simulink model "tesys"  (R2021b)
settings: Solver=ode45  StartTime=0  StopTime=inf  FixedStep=1000  RelTol=1e-3  EnableMultiTasking=on
settings Model: PauseTimes=0.0  Creator=ricker  LastModifiedBy=abbas
settings SolverCC: AlgebraicLoopSolver=TrustRegion
settings DataIOCC: LimitDataPoints=on  SaveFormat=Array  SignalLoggingSaveFormat=ModelDataLogs  ReturnWorkspaceOutputs=off  SignalLoggingName=sigsOut
settings OptimizationCC: LifeSpan=inf
settings DebuggingCC: SaveWithParameterizedLinksMsg=none  UnderspecifiedInitializationDetection=Classic  MergeDetectMultiDrivingBlocksExec=none  SignalResolutionControl=TryResolveAllWithWarning  MultiTaskDSMMsg=warning  MultiTaskCondExecSysMsg=none  SFUnexpectedBacktrackingDiag=warning  SFNoUnconditionalDefaultTransitionDiag=warning  SFExecutionAtInitializationDiag=none  SFMachineParentedDataDiag=warning  ArithmeticOperatorsInVariantConditions=warning
settings HardwareCC: ProdBitPerPointer=32  ProdBitPerSizeT=32  ProdBitPerPtrDiffT=32  ProdLargestAtomicFloat=None  ProdIntDivRoundTo=Undefined  ProdEndianess=Unspecified  ProdWordSize=32  ProdHWDeviceType=32-bit Generic  TargetUnknown=on
settings ModelReferenceCC: PropagateSignalLabelsOutOfModel=off
settings SFSimCC: SimUseLocalCustomCode=off  CustomCodeUndefinedFunction=UseInterfaceOnly
settings RTWCC: RTWUseLocalCustomCode=off
settings CodeAppCC: StateflowObjectComments=on
settings GRTTargetCC: TargetLangStandard=C89/C90 (ANSI)  CombineOutputUpdateFcns=off  GRTInterface=on
settings ConfigComp: CovMetricSettings=dw  CovSaveCumulativeToWorkspaceVar=on  CovSaveSingleToWorkspaceVar=on  CovExternalEMLEnable=off  CovSFcnEnable=off

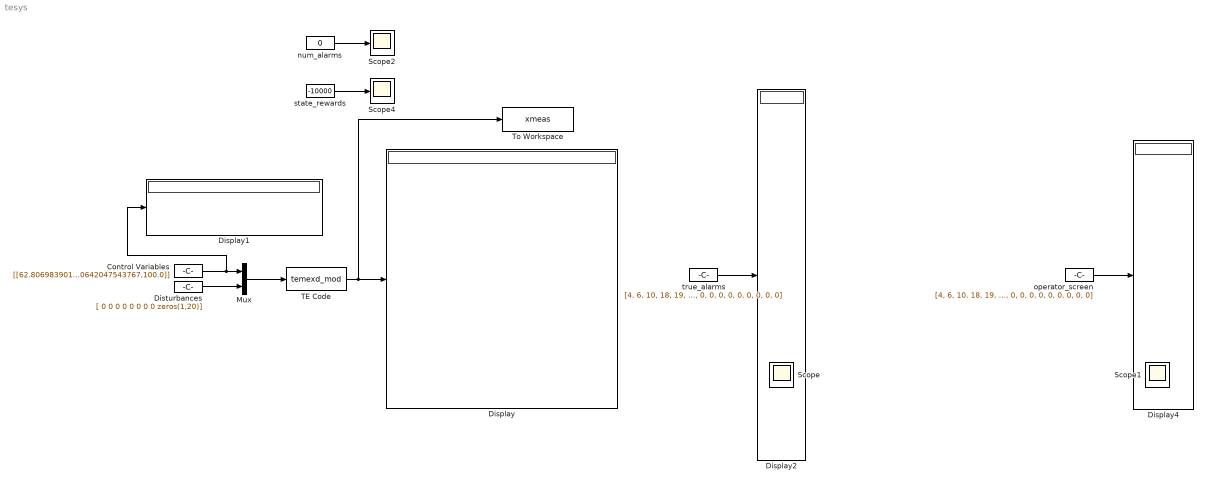
== system tesys ==
  Control Variables : Constant  Value=[[62.80698390115922,53.28670886135205,26.66217256336237,60.482853992876215,0.0,24.229300906565072,37.20819812809141,46.43052639510364,35.86532151232776,0.0,12.930642047543767,100.0]]
  Display{,1..2,4} (4 alike) : Display
  Disturbances : Constant  Value=[ 0 0 0 0 0 0 0 0 zeros(1,20)]
  Mux : Mux  Inputs=2
  Scope{,1..2,4} (4 alike) : Scope
  TE Code : S-Function  FunctionName=temexd_mod  SFunctionDeploymentMode=off  EnableBusSupport=off
  To Workspace : ToWorkspace  VariableName=xmeas  SampleTime=-1
      settings: MaxDataPoints=1
  num_alarms : Constant  Value=0
  operator_screen : Constant  Value=[4, 6, 10, 18, 19, 20, 22, 23, 24, 26, 28, 29, 30, 32, 36, 37, 0, 0, 0, 0, 0, 0, 0, 0, 0, 0, 0, 0, 0, 0, 0, 0, 0, 0, 0, 0, 0, 0]  VectorParams1D=off  OutDataTypeStr=double
  state_rewards : Constant  Value=-10000
  true_alarms : Constant  Value=[4, 6, 10, 18, 19, 20, 22, 23, 24, 26, 28, 29, 30, 32, 36, 37, 0, 0, 0, 0, 0, 0, 0, 0, 0, 0, 0, 0, 0, 0, 0, 0, 0, 0, 0, 0, 0, 0]  VectorParams1D=off  OutDataTypeStr=double
  wires:
  TE Code/1 -> To Workspace/1, Display/1
  Mux/1 -> TE Code/1
  Disturbances/1 -> Mux/2
  Control Variables/1 -> Display1/1, Mux/1
  true_alarms/1 -> Display2/1
  num_alarms/1 -> Scope2/1
  operator_screen/1 -> Display4/1
  state_rewards/1 -> Scope4/1
